simulink model "Sum3"  (R2020b)
settings: Solver=VariableStepAuto  StartTime=0.0  StopTime=20  FixedStep=1  RelTol=1e-3
settings Model: Creator=Aradhana desai  LastModifiedBy=Aradhana desai

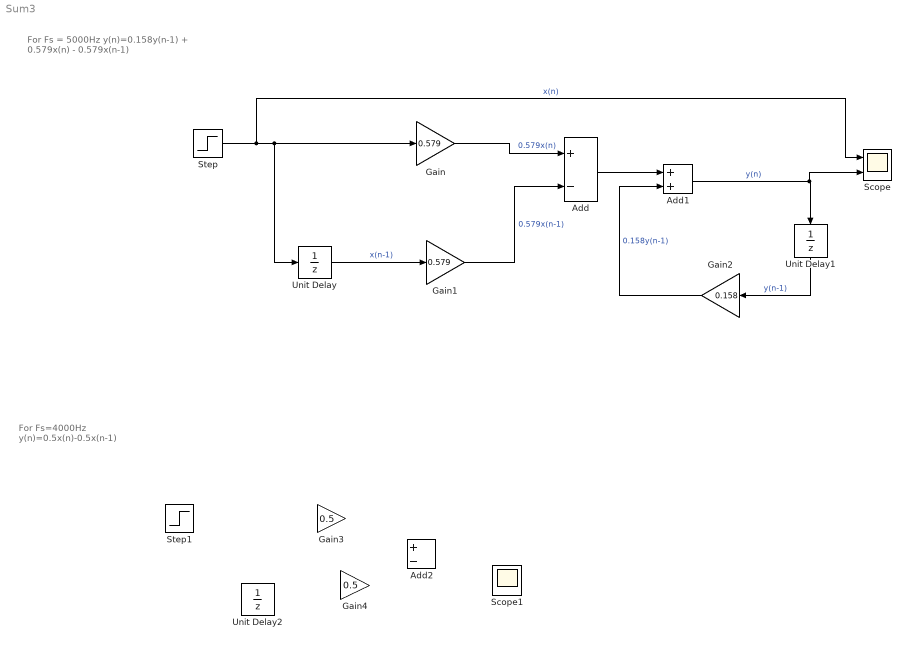
== system Sum3 ==
  note: For Fs=4000Hz
      | y(n)=0.5x(n)-0.5x(n-1)
  note: For Fs = 5000Hz
      | y(n)=0.158y(n-1) + 0.579x(n) - 0.579x(n-1)
  Add : Sum  Inputs=+-
  Add1 : Sum
  Add2 : Sum  Inputs=+-
  Gain : Gain  Gain=0.579
  Gain1 : Gain  Gain=0.579
  Gain2 : Gain  Gain=0.158
  Gain3 : Gain  Gain=0.5
  Gain4 : Gain  Gain=0.5
  Scope : Scope  NumInputPorts=2
  Scope1 : Scope
  Step : Step  SampleTime=0
  Step1 : Step  SampleTime=0
  Unit Delay : UnitDelay  SampleTime=-1  HasFrameUpgradeWarning=on
  Unit Delay1 : UnitDelay  SampleTime=-1  HasFrameUpgradeWarning=on
  Unit Delay2 : UnitDelay  SampleTime=-1  HasFrameUpgradeWarning=on
  wires:
  Unit Delay/1 -> Gain1/1  "x(n-1)"
  Gain1/1 -> Add/2  "0.579x(n-1)"
  Gain/1 -> Add/1  "0.579x(n)"
  Add/1 -> Add1/1
  Gain2/1 -> Add1/2  "0.158y(n-1)"
  Unit Delay1/1 -> Gain2/1  "y(n-1)"
  Add1/1 -> Scope/2, Unit Delay1/1  "y(n)"
  Step/1 -> Scope/1, Unit Delay/1, Gain/1  "x(n)"
